simulink model "closed_loop_system_monitoring"  (R2025b)
settings: Solver=FixedStepAuto  StartTime=0.0  StopTime=2  RelTol=1e-3
values from neighbouring files (symbols this model uses):
  A = [Ac 0*Ac ... (first row only)    [closed_loop_system.m]
  B = [Bc ... (first row only)    [closed_loop_system.m]
  C = [0 0 Cp]    [closed_loop_system.m]
  Ts = 1/100    (= 0.01)    [closed_loop_system.m]
(part 1 of 2)
settings Model: NumberOfSteps=5  Creator=elia  LastModifiedBy=elia

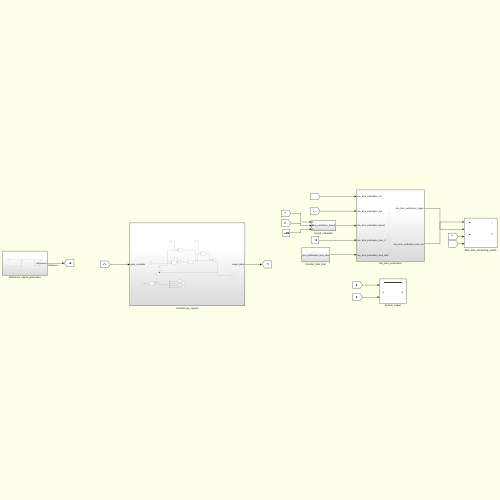
[thumbnail: Simulink's stored preview of the top-level diagram]
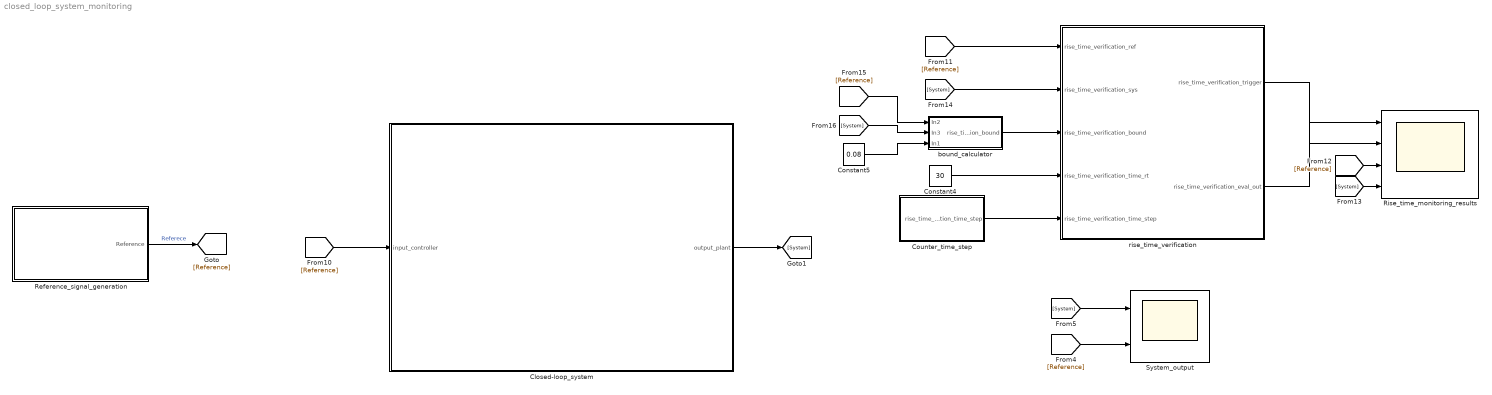
== system closed_loop_system_monitoring ==
  Closed-loop_system : Subsystem
  Constant4 : Constant  Value=30
  Constant5 : Constant  Value=0.08
  Counter_time_step : Subsystem
  Reference_signal_generation : Subsystem
  Rise_time_monitoring_results : Scope  NumInputPorts=4
      settings: ShowGrid=off  ActiveDisplayYMinimum=-0.12499999999999997  ActiveDisplayYMaximum=1.125  DataLoggingVariableName=ScopeData6
  System_output : Scope  NumInputPorts=2
      settings: ActiveDisplayYMinimum=-4.4796097220764581  ActiveDisplayYMaximum=1.9125014477904037
  bound_calculator : Subsystem
  rise_time_verification : Subsystem
  wires:
  Reference_signal_generation/1(Reference) -> [Reference]  "Referece"
  Closed-loop_system/1(output_plant) -> [System]
  [Reference] -> System_output/2
  [System] -> System_output/1
  [Reference] -> Closed-loop_system/1(input_controller)
  [System] -> rise_time_verification/2(rise_time_verification_sys)
  Constant4/1 -> rise_time_verification/4(rise_time_verification_time_rt)
  [System] -> Rise_time_monitoring_results/4
  rise_time_verification/2(rise_time_verification_eval_out) -> Rise_time_monitoring_results/1
  rise_time_verification/1(rise_time_verification_trigger) -> Rise_time_monitoring_results/2
  [Reference] -> Rise_time_monitoring_results/3
  Counter_time_step/1(rise_time_verification_time_step) -> rise_time_verification/5(rise_time_verification_time_step)
  [Reference] -> rise_time_verification/1(rise_time_verification_ref)
  Constant5/1 -> bound_calculator/3(In1)
  bound_calculator/1(rise_time_verification_bound) -> rise_time_verification/3(rise_time_verification_bound)
  [Reference] -> bound_calculator/1(In2)
  [System] -> bound_calculator/2(In3)

== system closed_loop_system_monitoring/Closed-loop_system ==
  input_controller : Inport
  Add : Sum  Inputs=-+
  Add1 : Sum
  Constant : Constant  Value=A
  Constant1 : Constant  Value=B
  Constant2 : Constant  Value=C
  Constant3 : Constant
  Constant4 : Constant  Value=0
  Constant5 : Constant  Value=0
  Constant6 : Constant  Value=0
  Matrix Multiply{,1..3} (4 alike) : Product  Multiplication=Matrix(*)
  Saturation : Subsystem
  Scope : Scope
  Transpose : Math  Operator=transpose
  Unit Delay : UnitDelay  SampleTime=-1  HasFrameUpgradeWarning=on
  Vector Concatenate : Concatenate  NumInputs=4
  output_plant : Outport
  wires:
  Constant/1 -> Matrix Multiply/1
  Constant1/1 -> Matrix Multiply1/1
  Saturation/1(Out1) -> Matrix Multiply1/2
  Add/1 -> Saturation/1(In1)
  Matrix Multiply2/1 -> Add/2
  Constant2/1 -> Matrix Multiply2/2
  Add1/1 -> Scope/1, Matrix Multiply3/2, Unit Delay/1
  Unit Delay/1 -> Matrix Multiply/2, Matrix Multiply2/1
  input_controller/1 -> Add/1
  Matrix Multiply1/1 -> Add1/1
  Matrix Multiply/1 -> Add1/2
  Vector Concatenate/1 -> Transpose/1
  Matrix Multiply3/1 -> output_plant/1
  Constant3/1 -> Vector Concatenate/3
  Constant4/1 -> Vector Concatenate/2
  Constant5/1 -> Vector Concatenate/1
  Constant6/1 -> Vector Concatenate/4
  Transpose/1 -> Matrix Multiply3/1

== system closed_loop_system_monitoring/Counter_time_step ==
  Add : Sum
  Constant4 : Constant  Value=0
  Constant5 : Constant
  Scope2 : Scope
      settings: ActiveDisplayYMinimum=-61.499999999999986  ActiveDisplayYMaximum=563.5  DataLoggingVariableName=ScopeData5
  Switch : Switch  Criteria=u2 ~= 0  SaturateOnIntegerOverflow=off  InputSameDT=off
  Unit Delay : UnitDelay  SampleTime=Ts  HasFrameUpgradeWarning=on
  Unit Delay1 : UnitDelay  SampleTime=Ts  HasFrameUpgradeWarning=on
  rise_time_verification_time_step : Outport
  wires:
  Switch/1 -> Add/1
  Add/1 -> Scope2/1, rise_time_verification_time_step/1, Unit Delay/1
  Constant5/1 -> Add/2
  Unit Delay1/1 -> Switch/2
  Unit Delay/1 -> Switch/3
  Constant4/1 -> Switch/1, Unit Delay1/1

== system closed_loop_system_monitoring/Reference_signal_generation ==
  Scope : Scope
      settings: ActiveDisplayYMinimum=0.9  ActiveDisplayYMaximum=1.1  DataLoggingVariableName=ScopeData4
  Step1 : Step  Time=0  Before=0.0  After=1.0  SampleTime=Ts
  Step2 : Step  Before=0.0  After=-3.0  SampleTime=Ts
  Sum : Sum  Inputs=|++
  Reference : Outport
  wires:
  Sum/1 -> Scope/1, Reference/1
  Step1/1 -> Sum/1  "input_1"
  Step2/1 -> Sum/2  "input_2"

== system closed_loop_system_monitoring/bound_calculator ==
  In2 : Inport
  In3 : Inport  Port=2
  In1 : Inport  Port=3
  Abs : Abs  SaturateOnIntegerOverflow=off
  Constant : Constant  Value=0
  Delay One Step : Delay  DelayLength=1  SampleTime=Ts
  Delay One Step1 : Delay  DelayLength=1  SampleTime=Ts
  Delay One Step2 : Delay  DelayLength=1  SampleTime=Ts
  Equal : RelationalOperator  Operator===  OutDataTypeStr=boolean  RndMeth=Simplest  InputSameDT=off
  NOT : Logic  Operator=NOT  IconShape=distinctive  AllPortsSameDT=off  OutDataTypeStr=boolean
  Product : Product
  Sum : Sum  Inputs=|+-
  Switch : Switch  Criteria=u2 > Threshold  SaturateOnIntegerOverflow=off  InputSameDT=off
  init : Switch  Criteria=u2 ~= 0  SaturateOnIntegerOverflow=off  InputSameDT=off
  rise_time_verification_bound : Outport
  wires:
  init/1 -> Delay One Step2/1, Product/1
  Constant/1 -> Delay One Step/1
  Delay One Step/1 -> init/2
  In2/1 -> Sum/1, Delay One Step1/1, Equal/1
  In3/1 -> Sum/2
  Sum/1 -> Abs/1
  Abs/1 -> Switch/1, init/1
  In1/1 -> Product/2
  Product/1 -> rise_time_verification_bound/1
  Equal/1 -> NOT/1
  NOT/1 -> Switch/2
  Delay One Step1/1 -> Equal/2
  Delay One Step2/1 -> Switch/3
  Switch/1 -> init/3

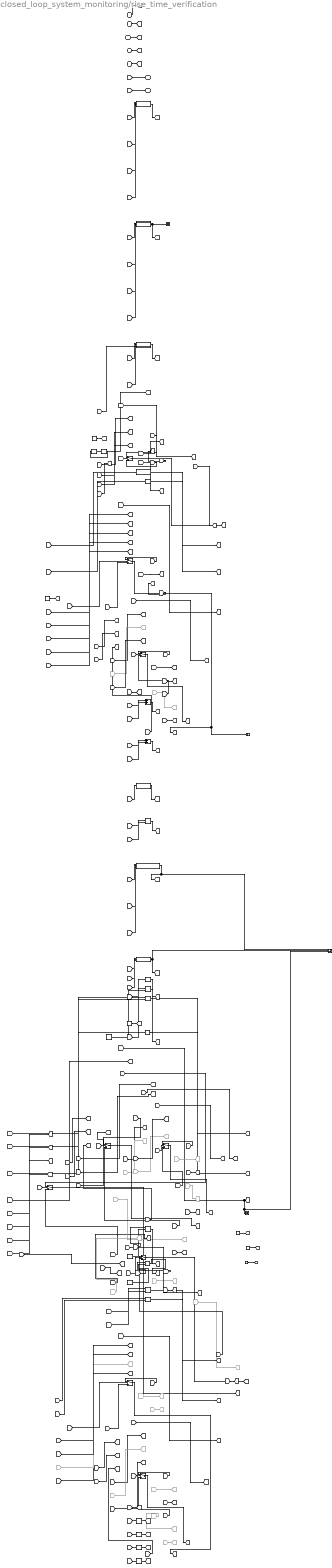
== system closed_loop_system_monitoring/rise_time_verification ==
  note: INIT time_step_reset
      | OK
  note: ITE time_step_reset
      | Guard+b_false OK
  note: ITE eval_out
      | OK
  note: INIT eval_out
      | Guard+init OK
  note: ITE eval : guard = pre trigger and pre eval
      | OK
  note: INIT trigger
      | OK
  note: ITE eval : guard = trigger
      | Guard+b_true OK
  note: ITE eval : guard = not ev_3v_T
      | OK
  note: ITE eval : guard = not ev_3v_F
      | OK
  rise_time_verification_ref : Inport  OutDataTypeStr=double
  rise_time_verification_sys : Inport  Port=2  OutDataTypeStr=double
  rise_time_verification_bound : Inport  Port=3  OutDataTypeStr=double
  rise_time_verification_time_rt : Inport  Port=4
  rise_time_verification_time_step : Inport  Port=5
  Arrow_xxrise_tim_1069005429_on_1_ni_18 : Delay  DelayLength=1  InitialCondition=1
  Constant : Constant  Value=0.5
  Constant1 : Constant  Value=1.0
  Constant2 : Constant  Value=0.25
  PRE_xxrise_time_verification_{2,11,13,22} (4 alike) : Delay  DelayLength=1  InitialCondition=0
  Scope : Scope
      settings: ActiveDisplayYMinimum=0.49776379028009476  ActiveDisplayYMaximum=0.51187913719672951  DataLoggingVariableName=ScopeData8
  Scope1 : Scope
      settings: ActiveDisplayYMinimum=-0.019336367279446723  ActiveDisplayYMaximum=0.04758303740367098  DataLoggingVariableName=ScopeData9
  Scope2 : Scope  NumInputPorts=3
      settings: ActiveDisplayYMinimum=-0.12499999999999997  ActiveDisplayYMaximum=1.125  DataLoggingVariableName=ScopeData10
  Scope3 : Scope
      settings: ActiveDisplayYMinimum=-50.249999999999986  ActiveDisplayYMaximum=452.25  DataLoggingVariableName=ScopeData11
  a_alse_xxrise_time_verification_7_out1 : Goto  Commented=on  GotoTag=a_alse_xxrise_time_verification_7
  a_alse_xxrise_time_verification_7_out2 : Goto  Commented=on  GotoTag=a_alse_xxrise_time_verification_7
  a_alse_xxrise_time_verification_7_out3 : Goto  Commented=on  GotoTag=a_alse_xxrise_time_verification_7
  a_lse_xxrise_time_verification_22_out1 : Goto  Commented=on  GotoTag=a_lse_xxrise_time_verification_22
  a_true_xxrise_time_verification_7_out{,1..2,4} (4 alike) : Goto  Commented=on  GotoTag=a_true_xxrise_time_verification_7
  absolute_value_call : Subsystem
  branch_13_IF : Switch  Criteria=u2 ~= 0  SaturateOnIntegerOverflow=off  InputSameDT=off
  branch_14_IF : Switch  Criteria=u2 ~= 0  SaturateOnIntegerOverflow=off  InputSameDT=off
  branch_15_IF : Switch  Criteria=u2 ~= 0  SaturateOnIntegerOverflow=off  InputSameDT=off
  branch_15_In2 : From  Commented=on  GotoTag=a_lse_xxrise_time_verification_22
  branch_15_branch_false_In1 : From  Commented=on  GotoTag=branch_15_xxrise_time_verification_22
  branch_15_xxrise_time_verification_22_out : Goto  Commented=on  GotoTag=branch_15_xxrise_time_verification_22
  branch_16_IF : Switch  Criteria=u2 ~= 0  SaturateOnIntegerOverflow=off  InputSameDT=off
  branch_17_IF : Switch  Criteria=u2 ~= 0  SaturateOnIntegerOverflow=off  InputSameDT=off
  branch_17_branch_false_In1 : From  Commented=on  GotoTag=branch_17_xxrise_time_verification_7
  branch_17_branch_true_In2 : From  Commented=on  GotoTag=branch_17_xxrise_time_verification_7
  branch_18_IF : Switch  Criteria=u2 ~= 0  SaturateOnIntegerOverflow=off  InputSameDT=off
  branch_18_In2 : From  Commented=on  GotoTag=a_true_xxrise_time_verification_7
  branch_18_branch_false_In1 : From  Commented=on  GotoTag=branch_18_xxrise_time_verification_7
  branch_18_branch_true_In1 : From  Commented=on  GotoTag=branch_18_xxrise_time_verification_7
  branch_18_xxrise_time_verification_7_out : Goto  Commented=on  GotoTag=branch_18_xxrise_time_verification_7
  branch_19_IF : Switch  Criteria=u2 ~= 0  SaturateOnIntegerOverflow=off  InputSameDT=off
  branch_19_In2 : From  Commented=on  GotoTag=a_alse_xxrise_time_verification_7
  branch_19_branch_false_In1 : From  Commented=on  GotoTag=branch_19_xxrise_time_verification_7
  branch_19_branch_true_In1 : From  Commented=on  GotoTag=branch_19_xxrise_time_verification_7
  branch_19_xxrise_time_verification_7_out : Goto  Commented=on  GotoTag=branch_19_xxrise_time_verification_7
  branch_20_IF : Switch  Criteria=u2 ~= 0  SaturateOnIntegerOverflow=off  InputSameDT=off
  branch_20_In3 : From  Commented=on  GotoTag=a_tion_xxrise_time_verification_7
  branch_20_branch_true_In1 : From  Commented=on  GotoTag=branch_20_eval
  branch_20_branch_true_eval_out : Goto  Commented=on  GotoTag=branch_20_branch_true_eval
  branch_20_xxrise_time_verification_7_out : Goto  Commented=on  GotoTag=branch_20_xxrise_time_verification_7
  branch_21_IF : Switch  Criteria=u2 ~= 0  SaturateOnIntegerOverflow=off  InputSameDT=off
  branch_21_In2 : From  Commented=on  GotoTag=a_alse_xxrise_time_verification_7
  branch_21_branch_false_In1 : From  Commented=on  GotoTag=branch_21_eval
  branch_21_branch_false_eval_out : Goto  Commented=on  GotoTag=branch_21_branch_false_eval
  branch_21_branch_true_In1 : From  Commented=on  GotoTag=branch_21_xxrise_time_verification_7
  branch_21_xxrise_time_verification_7_out : Goto  Commented=on  GotoTag=branch_21_xxrise_time_verification_7
  condition_R_call : Subsystem
  eventually_false_var_call : Subsystem
  eventually_true_var_call : Subsystem
  trigger_general_rt_call : Subsystem
  trigger_off_rise_time_call : Subsystem
  trigger_on_rise_time_call : Subsystem
  xxrise_tim_1069005429_on_1_ni_18_init : Constant  Value=0  OutDataTypeStr=boolean
  xxrise_time_verification_10_operator : Logic  Operator=NOT  AllPortsSameDT=off  OutDataTypeStr=boolean
  xxrise_time_verification_12_operator : RelationalOperator  Operator===  OutDataTypeStr=boolean  RndMeth=Simplest  InputSameDT=off
  xxrise_time_verification_12_rhs_2 : Constant  Value=0.5  OutDataTypeStr=double
  xxrise_time_verification_14_operator : Logic  AllPortsSameDT=off  OutDataTypeStr=boolean
  xxrise_time_verification_15_operator : Sum  Inputs=+-  OutDataTypeStr=double
  xxrise_time_verification_17_operator : RelationalOperator  Operator=<=  OutDataTypeStr=boolean  RndMeth=Simplest  InputSameDT=off
  xxrise_time_verification_18_operator : Sum  OutDataTypeStr=int32
  xxrise_time_verification_19_rhs : Constant  Value=0  OutDataTypeStr=Inherit: Inherit via back propagation
  xxrise_time_verification_21_operator : Logic  Operator=NOT  AllPortsSameDT=off  OutDataTypeStr=boolean
  xxrise_time_verification_24_rhs : Constant  Value=false  OutDataTypeStr=boolean
  xxrise_time_verification_3_operator : RelationalOperator  Operator===  OutDataTypeStr=boolean  RndMeth=Simplest  InputSameDT=off
  xxrise_time_verification_3_rhs_2 : Constant  Value=0.0  OutDataTypeStr=double
  xxrise_time_verification_4_operator : RelationalOperator  Operator===  OutDataTypeStr=boolean  RndMeth=Simplest  InputSameDT=off
  xxrise_time_verification_4_rhs_2 : Constant  Value=0.0  OutDataTypeStr=double
  xxrise_time_verification_5_operator : Logic  Operator=OR  AllPortsSameDT=off  OutDataTypeStr=boolean
  xxrise_time_verification_6_operator : Logic  AllPortsSameDT=off  OutDataTypeStr=boolean
  xxrise_time_verification_7_rhs : Constant  Value=0.0  OutDataTypeStr=double
  xxrise_time_verification_8_lhs : Goto  Commented=on  GotoTag=a_alse_xxrise_time_verification_8
  xxrise_time_verification_8_lhs2 : Goto  Commented=on  GotoTag=a_true_xxrise_time_verification_8
  xxrise_time_verification_8_rhs : From  Commented=on  GotoTag=branch_21_branch_false_eval
  xxrise_time_verification_8_rhs2 : From  Commented=on  GotoTag=branch_20_branch_true_eval
  xxrise_time_verification_9_operator : Logic  Operator=NOT  AllPortsSameDT=off  OutDataTypeStr=boolean
  rise_time_verification_trigger : Outport
  rise_time_verification_eval_out : Outport  Port=2
  wires:
  rise_time_verification_ref/1 -> [rise_time_verification_ref]
  rise_time_verification_sys/1 -> [rise_time_verification_sys]
  rise_time_verification_bound/1 -> [rise_time_verification_bound]
  rise_time_verification_time_rt/1 -> [rise_time_verification_time_rt]
  rise_time_verification_time_step/1 -> [rise_time_verification_time_step]
  [rise_time_verification_trigger] -> rise_time_verification_trigger/1
  [rise_time_verification_eval_out] -> rise_time_verification_eval_out/1
  trigger_on_rise_time_call/1(trigger_on_rise_time_trigger) -> [rise_time_verification_ev_ON]
  [a_ion_xxrise_time_verification_13] -> trigger_on_rise_time_call/1(trigger_on_rise_time_p_trigger)
  [rise_time_verification_ref] -> trigger_on_rise_time_call/2(trigger_on_rise_time_ref)
  [rise_time_verification_sys] -> trigger_on_rise_time_call/3(trigger_on_rise_time_sys)
  [rise_time_verification_bound] -> trigger_on_rise_time_call/4(trigger_on_rise_time_bound)
  trigger_off_rise_time_call/1(trigger_off_rise_time_trigger) -> [rise_time_verification_ev_OFF], Scope1/1
  [a_ion_xxrise_time_verification_13] -> trigger_off_rise_time_call/1(trigger_off_rise_time_p_trigger)
  [rise_time_verification_ref] -> trigger_off_rise_time_call/2(trigger_off_rise_time_ref)
  [rise_time_verification_sys] -> trigger_off_rise_time_call/3(trigger_off_rise_time_sys)
  [rise_time_verification_bound] -> trigger_off_rise_time_call/4(trigger_off_rise_time_bound)
  trigger_general_rt_call/1(trigger_general_rt_trigger_out) -> [a_ion_xxrise_time_verification_25]
  [rise_time_verification_ev_ON] -> trigger_general_rt_call/1(trigger_general_rt_ev_ON)
  [rise_time_verification_ev_OFF] -> trigger_general_rt_call/2(trigger_general_rt_ev_OFF)
  [rise_time_verification_ref] -> trigger_general_rt_call/3(trigger_general_rt_r)
  xxrise_time_verification_24_rhs/1 -> [a_ion_xxrise_time_verification_24]
  xxrise_tim_1069005429_on_1_ni_18_init/1 -> Arrow_xxrise_tim_1069005429_on_1_ni_18/1
  Arrow_xxrise_tim_1069005429_on_1_ni_18/1 -> [a_tion_xxrise_time_verification_1]
  [branch_13_xxrise_time_verification_26] -> [a_ion_xxrise_time_verification_26]
  branch_13_IF/1 -> [branch_13_xxrise_time_verification_26]
  [a_lse_xxrise_time_verification_26] -> branch_13_IF/3
  [a_rue_xxrise_time_verification_26] -> branch_13_IF/1
  [branch_13_xxrise_time_verification_1] -> branch_13_IF/2
  [a_ion_xxrise_time_verification_25] -> [branch_13_xxrise_time_verification_25]
  [a_ion_xxrise_time_verification_24] -> [branch_13_xxrise_time_verification_24]
  [a_tion_xxrise_time_verification_1] -> [branch_13_xxrise_time_verification_1]
  [a_lse_xxrise_time_verification_25] -> [a_lse_xxrise_time_verification_26]
  [branch_13_xxrise_time_verification_25] -> [a_lse_xxrise_time_verification_25]
  [a_rue_xxrise_time_verification_24] -> [a_rue_xxrise_time_verification_26]
  [branch_13_xxrise_time_verification_24] -> [a_rue_xxrise_time_verification_24]
  [a_ion_xxrise_time_verification_26] -> [rise_time_verification_trigger]
  condition_R_call/1(condition_R_const_deriv) -> [a_ion_xxrise_time_verification_20]
  [rise_time_verification_ref] -> condition_R_call/1(condition_R_r)
  xxrise_time_verification_21_operator/1 -> [a_ion_xxrise_time_verification_21]
  [a_ion_xxrise_time_verification_20] -> xxrise_time_verification_21_operator/1
  xxrise_time_verification_19_rhs/1 -> [a_ion_xxrise_time_verification_19]
  [branch_14_xxrise_time_verification_23] -> [a_ion_xxrise_time_verification_23]
  branch_14_IF/1 -> Scope3/1, [branch_14_xxrise_time_verification_23]
  [a_lse_xxrise_time_verification_23_b_14_in] -> branch_14_IF/3
  [a_rue_xxrise_time_verification_23_b_14_init] -> branch_14_IF/1
  [branch_14_xxrise_time_verification_1] -> branch_14_IF/2
  [rise_time_verification_time_step] -> [branch_14_time_step]
  [a_ion_xxrise_time_verification_22] -> [branch_14_xxrise_time_verification_22]
  [a_ion_xxrise_time_verification_21] -> [branch_14_xxrise_time_verification_21]
  [a_ion_xxrise_time_verification_19] -> [branch_14_xxrise_time_verification_19]
  [a_tion_xxrise_time_verification_1] -> [branch_14_xxrise_time_verification_1]
  [branch_15_time_step] -> [branch_15_branch_true_time_step]
  [branch_15_branch_true_time_step] -> [a_rue_xxrise_time_verification_23]
  branch_15_branch_false_In1/1 -> a_lse_xxrise_time_verification_22_out1/1
  [a_lse_xxrise_time_verification_22_b_15_f] -> [a_lse_xxrise_time_verification_23]
  [a_lse_xxrise_time_verification_21] -> [branch_15_xxrise_time_verification_21]
  branch_15_In2/1 -> branch_15_xxrise_time_verification_22_out/1
  [branch_14_branch_false_time_step] -> [branch_15_time_step]
  [branch_15_xxrise_time_verification_21] -> branch_15_IF/2
  [a_rue_xxrise_time_verification_23] -> branch_15_IF/1
  [a_lse_xxrise_time_verification_23] -> branch_15_IF/3
  branch_15_IF/1 -> [branch_15_xxrise_time_verification_23]
  [branch_15_xxrise_time_verification_23] -> [a_lse_xxrise_time_verification_23_b_14_in]
  [branch_14_time_step] -> [branch_14_branch_false_time_step]
  [branch_14_xxrise_time_verification_22] -> [a_lse_xxrise_time_verification_22_b_15_f]
  [branch_14_xxrise_time_verification_21] -> [a_lse_xxrise_time_verification_21]
  [a_rue_xxrise_time_verification_19] -> [a_rue_xxrise_time_verification_23_b_14_init]
  [branch_14_xxrise_time_verification_19] -> [a_rue_xxrise_time_verification_19]
  [a_ion_xxrise_time_verification_23] -> [rise_time_verification_time_step_reset]
  xxrise_time_verification_18_operator/1 -> [a_ion_xxrise_time_verification_18]
  [rise_time_verification_time_rt] -> xxrise_time_verification_18_operator/1
  [rise_time_verification_time_step_reset] -> xxrise_time_verification_18_operator/2
  xxrise_time_verification_15_operator/1 -> [a_ion_xxrise_time_verification_15]
  [rise_time_verification_sys] -> xxrise_time_verification_15_operator/1
  [rise_time_verification_ref] -> xxrise_time_verification_15_operator/2
  absolute_value_call/1(absolute_value_abs) -> [a_ion_xxrise_time_verification_16]
  [a_ion_xxrise_time_verification_15] -> absolute_value_call/1(absolute_value_x)
  xxrise_time_verification_17_operator/1 -> [a_ion_xxrise_time_verification_17]
  [a_ion_xxrise_time_verification_16] -> xxrise_time_verification_17_operator/1
  [rise_time_verification_bound] -> xxrise_time_verification_17_operator/2
  eventually_true_var_call/1(eventually_true_var_output_ev_true) -> [rise_time_verification_eventually_3v_T], Scope2/1
  [rise_time_verification_time_step_reset] -> eventually_true_var_call/1(eventually_true_var_a)
  [a_ion_xxrise_time_verification_18] -> eventually_true_var_call/2(eventually_true_var_b)
  [a_ion_xxrise_time_verification_17] -> eventually_true_var_call/3(eventually_true_var_phi)
  eventually_false_var_call/1(eventually_false_var_output_ev_false) -> Scope2/2, [rise_time_verification_eventually_3v_F]
  [rise_time_verification_time_step_reset] -> eventually_false_var_call/1(eventually_false_var_a)
  [a_ion_xxrise_time_verification_18] -> eventually_false_var_call/2(eventually_false_var_b)
  [a_ion_xxrise_time_verification_17] -> eventually_false_var_call/3(eventually_false_var_phi)
  xxrise_time_verification_9_operator/1 -> [a_tion_xxrise_time_verification_9]
  [rise_time_verification_eventually_3v_T] -> xxrise_time_verification_9_operator/1
  xxrise_time_verification_7_rhs/1 -> [a_tion_xxrise_time_verification_7]
  xxrise_time_verification_12_operator/1 -> [a_ion_xxrise_time_verification_12]
  [a_ion_xxrise_time_verification_11] -> xxrise_time_verification_12_operator/1
  xxrise_time_verification_12_rhs_2/1 -> xxrise_time_verification_12_operator/2
  xxrise_time_verification_14_operator/1 -> [a_ion_xxrise_time_verification_14]
  [a_ion_xxrise_time_verification_13] -> xxrise_time_verification_14_operator/1
  [a_ion_xxrise_time_verification_12] -> xxrise_time_verification_14_operator/2
  xxrise_time_verification_10_operator/1 -> [a_ion_xxrise_time_verification_10]
  [rise_time_verification_eventually_3v_F] -> xxrise_time_verification_10_operator/1
  [branch_16_eval] -> Scope2/3, Scope/1, [rise_time_verification_eval]
  branch_16_IF/1 -> [branch_16_eval]
  [branch_16_branch_false_eval] -> branch_16_IF/3
  [branch_16_branch_true_eval] -> branch_16_IF/1
  [branch_16_trigger] -> branch_16_IF/2
  [rise_time_verification_trigger] -> [branch_16_trigger]
  [a_tion_xxrise_time_verification_9] -> [branch_16_xxrise_time_verification_9]
  [a_tion_xxrise_time_verification_7] -> [branch_16_xxrise_time_verification_7]
  [a_ion_xxrise_time_verification_14] -> [branch_16_xxrise_time_verification_14]
  [a_ion_xxrise_time_verification_10] -> [branch_16_xxrise_time_verification_10]
  branch_19_branch_true_In1/1 -> a_true_xxrise_time_verification_7_out/1
  [const_1_0] -> [branch_19_branch_true_eval]
  branch_19_branch_false_In1/1 -> a_alse_xxrise_time_verification_7_out1/1
  [a_alse_xxrise_time_verification_7] -> [branch_19_branch_false_eval]
  [a_lse_xxrise_time_verification_14] -> [branch_19_xxrise_time_verification_14]
  branch_19_In2/1 -> branch_19_xxrise_time_verification_7_out/1
  [branch_19_xxrise_time_verification_14] -> branch_19_IF/2
  [branch_19_branch_true_eval] -> branch_19_IF/1
  [branch_19_branch_false_eval] -> branch_19_IF/3
  branch_19_IF/1 -> [branch_19_eval]
  [branch_19_eval] -> [branch_16_branch_false_eval]
  [branch_16_xxrise_time_verification_7] -> [a_alse_xxrise_time_verification_7_b_18_F]
  [branch_16_xxrise_time_verification_14] -> [a_lse_xxrise_time_verification_14]
  [branch_17_xxrise_time_verification_10] -> [a_rue_xxrise_time_verification_10]
  branch_17_branch_true_In2/1 -> a_true_xxrise_time_verification_7_out2/1
  [branch_18_eval] -> [branch_17_branch_true_eval]
  branch_18_IF/1 -> [branch_18_eval]
  [branch_18_branch_false_eval] -> branch_18_IF/3
  [branch_18_branch_true_eval] -> branch_18_IF/1
  [branch_18_xxrise_time_verification_10] -> branch_18_IF/2
  branch_18_In2/1 -> branch_18_xxrise_time_verification_7_out/1
  [a_rue_xxrise_time_verification_10] -> [branch_18_xxrise_time_verification_10]
  [a_alse_xxrise_time_verification_7_b_18_F] -> [branch_18_branch_false_eval]
  branch_18_branch_false_In1/1 -> a_alse_xxrise_time_verification_7_out3/1
  [const_0_5] -> [branch_18_branch_true_eval]
  branch_18_branch_true_In1/1 -> a_true_xxrise_time_verification_7_out1/1
  branch_17_branch_false_In1/1 -> a_alse_xxrise_time_verification_7_out2/1
  [const_1_0] -> [branch_17_branch_false_eval]
  [a_rue_xxrise_time_verification_10_guard_b_18] -> [branch_17_xxrise_time_verification_10]
  [a_true_xxrise_time_verification_7] -> [branch_17_xxrise_time_verification_7]
  [a_true_xxrise_time_verification_9] -> [branch_17_xxrise_time_verification_9]
  [branch_17_xxrise_time_verification_9] -> branch_17_IF/2
  [branch_17_branch_true_eval] -> branch_17_IF/1
  [branch_17_branch_false_eval] -> branch_17_IF/3
  branch_17_IF/1 -> [branch_17_eval]
  [branch_17_eval] -> [branch_16_branch_true_eval]
  [branch_16_xxrise_time_verification_9] -> [a_true_xxrise_time_verification_9]
  [branch_16_xxrise_time_verification_7] -> [a_true_xxrise_time_verification_7]
  [branch_16_xxrise_time_verification_10] -> [a_rue_xxrise_time_verification_10_guard_b_18]
  xxrise_time_verification_4_operator/1 -> [a_tion_xxrise_time_verification_4]
  [rise_time_verification_eval] -> xxrise_time_verification_4_operator/1
  xxrise_time_verification_4_rhs_2/1 -> xxrise_time_verification_4_operator/2
  xxrise_time_verification_3_operator/1 -> [a_tion_xxrise_time_verification_3]
  [a_tion_xxrise_time_verification_2] -> xxrise_time_verification_3_operator/1
  xxrise_time_verification_3_rhs_2/1 -> xxrise_time_verification_3_operator/2
  xxrise_time_verification_5_operator/1 -> [a_tion_xxrise_time_verification_5]
  [a_tion_xxrise_time_verification_4] -> xxrise_time_verification_5_operator/1
  [a_tion_xxrise_time_verification_3] -> xxrise_time_verification_5_operator/2
  xxrise_time_verification_6_operator/1 -> [a_tion_xxrise_time_verification_6]
  [rise_time_verification_trigger] -> xxrise_time_verification_6_operator/1
  [a_tion_xxrise_time_verification_5] -> xxrise_time_verification_6_operator/2
  [branch_20_xxrise_time_verification_8] -> [a_tion_xxrise_time_verification_8]
  branch_20_IF/1 -> [branch_20_xxrise_time_verification_8]
  [a_alse_xxrise_time_verification_8_b_21_F] -> branch_20_IF/3
  [rise_time_verification_eval] -> branch_20_IF/1
  [branch_20_xxrise_time_verification_1] -> branch_20_IF/2
  [rise_time_verification_eval] -> [branch_20_eval]
  branch_20_In3/1 -> branch_20_xxrise_time_verification_7_out/1
  [a_tion_xxrise_time_verification_6] -> [branch_20_xxrise_time_verification_6]
  [a_tion_xxrise_time_verification_1] -> [branch_20_xxrise_time_verification_1]
  branch_21_branch_true_In1/1 -> a_true_xxrise_time_verification_7_out4/1
  [a_true_xxrise_time_verification_7] -> [a_true_xxrise_time_verification_8_b_21_in]
  branch_21_branch_false_In1/1 -> branch_21_branch_false_eval_out/1
  xxrise_time_verification_8_rhs/1 -> xxrise_time_verification_8_lhs/1
  [a_alse_xxrise_time_verification_6] -> [branch_21_xxrise_time_verification_6]
  branch_21_In2/1 -> branch_21_xxrise_time_verification_7_out/1
  [branch_20_branch_false_eval] -> [branch_21_eval]
  [branch_21_xxrise_time_verification_6] -> branch_21_IF/2
  [a_true_xxrise_time_verification_8_b_21_in] -> branch_21_IF/1
  [rise_time_verification_eval] -> branch_21_IF/3
  branch_21_IF/1 -> [branch_21_xxrise_time_verification_8]
  [branch_21_xxrise_time_verification_8] -> [a_alse_xxrise_time_verification_8_b_21_F]
  [branch_20_eval] -> [branch_20_branch_false_eval]
  [const_0_25] -> [a_alse_xxrise_time_verification_7]
  [branch_20_xxrise_time_verification_6] -> [a_alse_xxrise_time_verification_6]
  xxrise_time_verification_8_rhs2/1 -> xxrise_time_verification_8_lhs2/1
  branch_20_branch_true_In1/1 -> branch_20_branch_true_eval_out/1
  [a_tion_xxrise_time_verification_8] -> [rise_time_verification_eval_out]
  [rise_time_verification_time_step_reset] -> PRE_xxrise_time_verification_22/1
  PRE_xxrise_time_verification_22/1 -> [a_ion_xxrise_time_verification_22]
  [rise_time_verification_eval_out] -> PRE_xxrise_time_verification_2/1
  PRE_xxrise_time_verification_2/1 -> [a_tion_xxrise_time_verification_2]
  [rise_time_verification_trigger] -> PRE_xxrise_time_verification_13/1
  PRE_xxrise_time_verification_13/1 -> [a_ion_xxrise_time_verification_13]
  [rise_time_verification_eval] -> PRE_xxrise_time_verification_11/1
  PRE_xxrise_time_verification_11/1 -> [a_ion_xxrise_time_verification_11]
  Constant/1 -> [const_0_5]
  Constant1/1 -> [const_1_0]
  Constant2/1 -> [const_0_25]

== system closed_loop_system_monitoring/Closed-loop_system/Saturation ==
  In1 : Inport
  Constant : Constant  Value=1.0
  Constant1 : Constant  Value=-1.0
  Switch : Switch  Criteria=u2 > Threshold  Threshold=1.0  SaturateOnIntegerOverflow=off  InputSameDT=off
  Switch1 : Switch  Criteria=u2 > Threshold  Threshold=-1.0  SaturateOnIntegerOverflow=off  InputSameDT=off
  Out1 : Outport
  wires:
  Constant1/1 -> Switch1/3
  Constant/1 -> Switch/1
  Switch/1 -> Switch1/2, Switch1/1
  Switch1/1 -> Out1/1
  In1/1 -> Switch/2, Switch/3

== system closed_loop_system_monitoring/rise_time_verification/absolute_value_call ==
  absolute_value_x : Inport  OutDataTypeStr=double
  branch_8_IF : Switch  Criteria=u2 ~= 0  SaturateOnIntegerOverflow=off  InputSameDT=off
  xxabsolute_value_1_operator : RelationalOperator  OutDataTypeStr=boolean  RndMeth=Simplest  InputSameDT=off
  xxabsolute_value_1_rhs_2 : Constant  Value=0.0  OutDataTypeStr=double
  xxabsolute_value_2_operator : Gain  Gain=-1  OutDataTypeStr=double
  absolute_value_abs : Outport
  wires:
  [branch_8_x] -> [branch_8_branch_true_x]
  [branch_8_branch_true_x] -> [branch_8_branch_true_abs]
  [branch_8_xxabsolute_value_2] -> [branch_8_branch_false_xxabsolute_value_2]
  [branch_8_branch_false_xxabsolute_value_2] -> [branch_8_branch_false_abs]
  [absolute_value_xxabsolute_value_1] -> [branch_8_xxabsolute_value_1]
  [absolute_value_xxabsolute_value_2] -> [branch_8_xxabsolute_value_2]
  [absolute_value_x] -> [branch_8_x]
  [branch_8_xxabsolute_value_1] -> branch_8_IF/2
  [branch_8_branch_true_abs] -> branch_8_IF/1
  [branch_8_branch_false_abs] -> branch_8_IF/3
  branch_8_IF/1 -> [branch_8_abs]
  [branch_8_abs] -> [absolute_value_abs]
  xxabsolute_value_1_rhs_2/1 -> xxabsolute_value_1_operator/2
  [absolute_value_x] -> xxabsolute_value_1_operator/1
  xxabsolute_value_1_operator/1 -> [absolute_value_xxabsolute_value_1]
  [absolute_value_x] -> xxabsolute_value_2_operator/1
  xxabsolute_value_2_operator/1 -> [absolute_value_xxabsolute_value_2]
  [absolute_value_abs] -> absolute_value_abs/1
  absolute_value_x/1 -> [absolute_value_x]

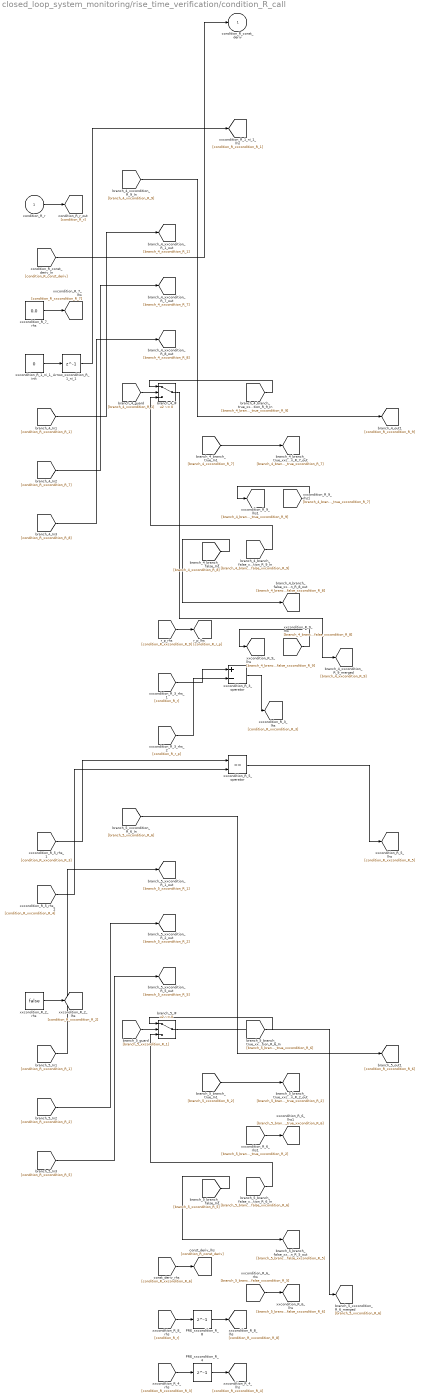
== system closed_loop_system_monitoring/rise_time_verification/condition_R_call ==
  condition_R_r : Inport  OutDataTypeStr=double
  Arrow_xxcondition_R_1_ni_1 : Delay  DelayLength=1  InitialCondition=1
  PRE_xxcondition_R_4 : Delay  DelayLength=1  InitialCondition=0
  PRE_xxcondition_R_8 : Delay  DelayLength=1  InitialCondition=0
  branch_4_IF : Switch  Criteria=u2 ~= 0  SaturateOnIntegerOverflow=off  InputSameDT=off
  branch_5_IF : Switch  Criteria=u2 ~= 0  SaturateOnIntegerOverflow=off  InputSameDT=off
  xxcondition_R_1_ni_1_init : Constant  Value=0  OutDataTypeStr=boolean
  xxcondition_R_2_rhs : Constant  Value=false  OutDataTypeStr=boolean
  xxcondition_R_3_operator : Sum  Inputs=+-  OutDataTypeStr=double
  xxcondition_R_5_operator : RelationalOperator  Operator===  OutDataTypeStr=boolean  RndMeth=Simplest  InputSameDT=off
  xxcondition_R_7_rhs : Constant  Value=0.0  OutDataTypeStr=double
  condition_R_const_deriv : Outport
  wires:
  PRE_xxcondition_R_4/1 -> [condition_R_xxcondition_R_4]
  [condition_R_xxcondition_R_3] -> PRE_xxcondition_R_4/1
  PRE_xxcondition_R_8/1 -> [condition_R_xxcondition_R_8]
  [condition_R_r] -> PRE_xxcondition_R_8/1
  [condition_R_xxcondition_R_6] -> [condition_R_const_deriv]
  [branch_5_xxcondition_R_2] -> [branch_5_branch_true_xxcondition_R_2]
  [branch_5_branch_true_xxcondition_R_2] -> [branch_5_branch_true_xxcondition_R_6]
  [branch_5_xxcondition_R_5] -> [branch_5_branch_false_xxcondition_R_5]
  [branch_5_branch_false_xxcondition_R_5] -> [branch_5_branch_false_xxcondition_R_6]
  [condition_R_xxcondition_R_1] -> [branch_5_xxcondition_R_1]
  [condition_R_xxcondition_R_2] -> [branch_5_xxcondition_R_2]
  [condition_R_xxcondition_R_5] -> [branch_5_xxcondition_R_5]
  [branch_5_xxcondition_R_1] -> branch_5_IF/2
  [branch_5_branch_true_xxcondition_R_6] -> branch_5_IF/1
  [branch_5_branch_false_xxcondition_R_6] -> branch_5_IF/3
  branch_5_IF/1 -> [branch_5_xxcondition_R_6]
  [branch_5_xxcondition_R_6] -> [condition_R_xxcondition_R_6]
  xxcondition_R_2_rhs/1 -> [condition_R_xxcondition_R_2]
  [condition_R_xxcondition_R_4] -> xxcondition_R_5_operator/2
  [condition_R_xxcondition_R_3] -> xxcondition_R_5_operator/1
  xxcondition_R_5_operator/1 -> [condition_R_xxcondition_R_5]
  [condition_R_r_p] -> xxcondition_R_3_operator/2
  [condition_R_r] -> xxcondition_R_3_operator/1
  xxcondition_R_3_operator/1 -> [condition_R_xxcondition_R_3]
  [condition_R_xxcondition_R_9] -> [condition_R_r_p]
  [branch_4_xxcondition_R_7] -> [branch_4_branch_true_xxcondition_R_7]
  [branch_4_branch_true_xxcondition_R_7] -> [branch_4_branch_true_xxcondition_R_9]
  [branch_4_xxcondition_R_8] -> [branch_4_branch_false_xxcondition_R_8]
  [branch_4_branch_false_xxcondition_R_8] -> [branch_4_branch_false_xxcondition_R_9]
  [condition_R_xxcondition_R_1] -> [branch_4_xxcondition_R_1]
  [condition_R_xxcondition_R_7] -> [branch_4_xxcondition_R_7]
  [condition_R_xxcondition_R_8] -> [branch_4_xxcondition_R_8]
  [branch_4_xxcondition_R_1] -> branch_4_IF/2
  [branch_4_branch_true_xxcondition_R_9] -> branch_4_IF/1
  [branch_4_branch_false_xxcondition_R_9] -> branch_4_IF/3
  branch_4_IF/1 -> [branch_4_xxcondition_R_9]
  [branch_4_xxcondition_R_9] -> [condition_R_xxcondition_R_9]
  Arrow_xxcondition_R_1_ni_1/1 -> [condition_R_xxcondition_R_1]
  xxcondition_R_1_ni_1_init/1 -> Arrow_xxcondition_R_1_ni_1/1
  xxcondition_R_7_rhs/1 -> [condition_R_xxcondition_R_7]
  [condition_R_const_deriv] -> condition_R_const_deriv/1
  condition_R_r/1 -> [condition_R_r]

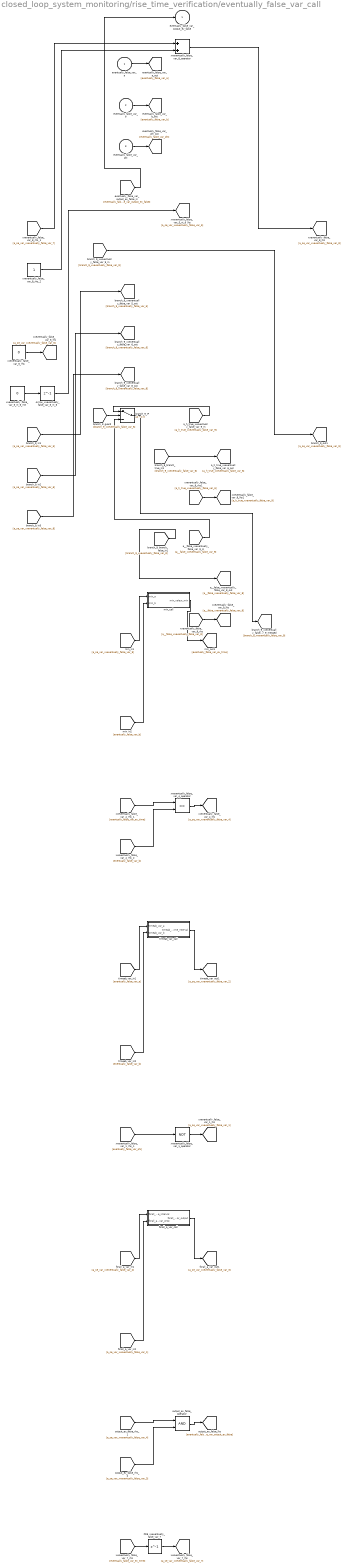
== system closed_loop_system_monitoring/rise_time_verification/eventually_false_var_call ==
  eventually_false_var_a : Inport
  eventually_false_var_b : Inport  Port=2
  eventually_false_var_phi : Inport  Port=3  OutDataTypeStr=boolean
  Arrow_xxeventually_false_var_5_ni_6 : Delay  DelayLength=1  InitialCondition=1
  PRE_xxeventually_false_var_7 : Delay  DelayLength=1  InitialCondition=0
  branch_9_IF : Switch  Criteria=u2 ~= 0  SaturateOnIntegerOverflow=off  InputSameDT=off
  forall_a_var_call : Subsystem
  min_call : Subsystem
  output_ev_false_operator : Logic  AllPortsSameDT=off  OutDataTypeStr=boolean
  timeab_var_call : Subsystem
  xxeventually_false_var_1_operator : Logic  Operator=NOT  AllPortsSameDT=off  OutDataTypeStr=boolean
  xxeventually_false_var_4_operator : RelationalOperator  Operator===  OutDataTypeStr=boolean  RndMeth=Simplest  InputSameDT=off
  xxeventually_false_var_5_ni_6_init : Constant  Value=0  OutDataTypeStr=boolean
  xxeventually_false_var_6_rhs : Constant  Value=0  OutDataTypeStr=Inherit: Inherit via back propagation
  xxeventually_false_var_8_operator : Sum  OutDataTypeStr=int32
  xxeventually_false_var_8_rhs_2 : Constant  OutDataTypeStr=int32
  eventually_false_var_output_ev_false : Outport
  wires:
  PRE_xxeventually_false_var_7/1 -> [a_se_var_xxeventually_false_var_7]
  [eventually_false_var_ev_time] -> PRE_xxeventually_false_var_7/1
  [a_se_var_xxeventually_false_var_3] -> output_ev_false_operator/2
  [a_se_var_xxeventually_false_var_4] -> output_ev_false_operator/1
  output_ev_false_operator/1 -> [eventually_false_var_output_ev_false]
  [a_se_var_xxeventually_false_var_1] -> forall_a_var_call/2(forall_a_var_prop)
  [a_se_var_xxeventually_false_var_2] -> forall_a_var_call/1(forall_a_var_inside_time_interval)
  forall_a_var_call/1(forall_a_var_output) -> [a_se_var_xxeventually_false_var_3]
  [eventually_false_var_phi] -> xxeventually_false_var_1_operator/1
  xxeventually_false_var_1_operator/1 -> [a_se_var_xxeventually_false_var_1]
  [eventually_false_var_b] -> timeab_var_call/2(timeab_var_b)
  [eventually_false_var_a] -> timeab_var_call/1(timeab_var_a)
  timeab_var_call/1(timeab_var_inside_time_interval) -> [a_se_var_xxeventually_false_var_2]
  [eventually_false_var_b] -> xxeventually_false_var_4_operator/2
  [eventually_false_var_ev_time] -> xxeventually_false_var_4_operator/1
  xxeventually_false_var_4_operator/1 -> [a_se_var_xxeventually_false_var_4]
  [eventually_false_var_b] -> min_call/2(min_b)
  [a_se_var_xxeventually_false_var_9] -> min_call/1(min_a)
  min_call/1(min_valeur_min) -> [eventually_false_var_ev_time]
  [branch_9_xxeventually_false_var_6] -> [a_h_true_xxeventually_false_var_6]
  [a_h_true_xxeventually_false_var_6] -> [a_h_true_xxeventually_false_var_9]
  [branch_9_xxeventually_false_var_8] -> [a__false_xxeventually_false_var_8]
  [a__false_xxeventually_false_var_8] -> [a__false_xxeventually_false_var_9]
  [a_se_var_xxeventually_false_var_5] -> [branch_9_xxeventually_false_var_5]
  [a_se_var_xxeventually_false_var_6] -> [branch_9_xxeventually_false_var_6]
  [a_se_var_xxeventually_false_var_8] -> [branch_9_xxeventually_false_var_8]
  [branch_9_xxeventually_false_var_5] -> branch_9_IF/2
  [a_h_true_xxeventually_false_var_9] -> branch_9_IF/1
  [a__false_xxeventually_false_var_9] -> branch_9_IF/3
  branch_9_IF/1 -> [branch_9_xxeventually_false_var_9]
  [branch_9_xxeventually_false_var_9] -> [a_se_var_xxeventually_false_var_9]
  Arrow_xxeventually_false_var_5_ni_6/1 -> [a_se_var_xxeventually_false_var_5]
  xxeventually_false_var_5_ni_6_init/1 -> Arrow_xxeventually_false_var_5_ni_6/1
  xxeventually_false_var_6_rhs/1 -> [a_se_var_xxeventually_false_var_6]
  xxeventually_false_var_8_rhs_2/1 -> xxeventually_false_var_8_operator/2
  [a_se_var_xxeventually_false_var_7] -> xxeventually_false_var_8_operator/1
  xxeventually_false_var_8_operator/1 -> [a_se_var_xxeventually_false_var_8]
  [eventually_false_var_output_ev_false] -> eventually_false_var_output_ev_false/1
  eventually_false_var_phi/1 -> [eventually_false_var_phi]
  eventually_false_var_b/1 -> [eventually_false_var_b]
  eventually_false_var_a/1 -> [eventually_false_var_a]

== system closed_loop_system_monitoring/rise_time_verification/eventually_true_var_call ==
  eventually_true_var_a : Inport
  eventually_true_var_b : Inport  Port=2
  eventually_true_var_phi : Inport  Port=3  OutDataTypeStr=boolean
  exist_var_call : Subsystem
  timeab_var_call : Subsystem
  eventually_true_var_output_ev_true : Outport
  wires:
  [eventually_true_var_phi] -> exist_var_call/2(exist_var_prop)
  [eventually_true_var_xxeventually_true_var_1] -> exist_var_call/1(exist_var_inside_time_interval)
  exist_var_call/1(exist_var_output) -> [eventually_true_var_output_ev_true]
  [eventually_true_var_b] -> timeab_var_call/2(timeab_var_b)
  [eventually_true_var_a] -> timeab_var_call/1(timeab_var_a)
  timeab_var_call/1(timeab_var_inside_time_interval) -> [eventually_true_var_xxeventually_true_var_1]
  [eventually_true_var_output_ev_true] -> eventually_true_var_output_ev_true/1
  eventually_true_var_phi/1 -> [eventually_true_var_phi]
  eventually_true_var_b/1 -> [eventually_true_var_b]
  eventually_true_var_a/1 -> [eventually_true_var_a]

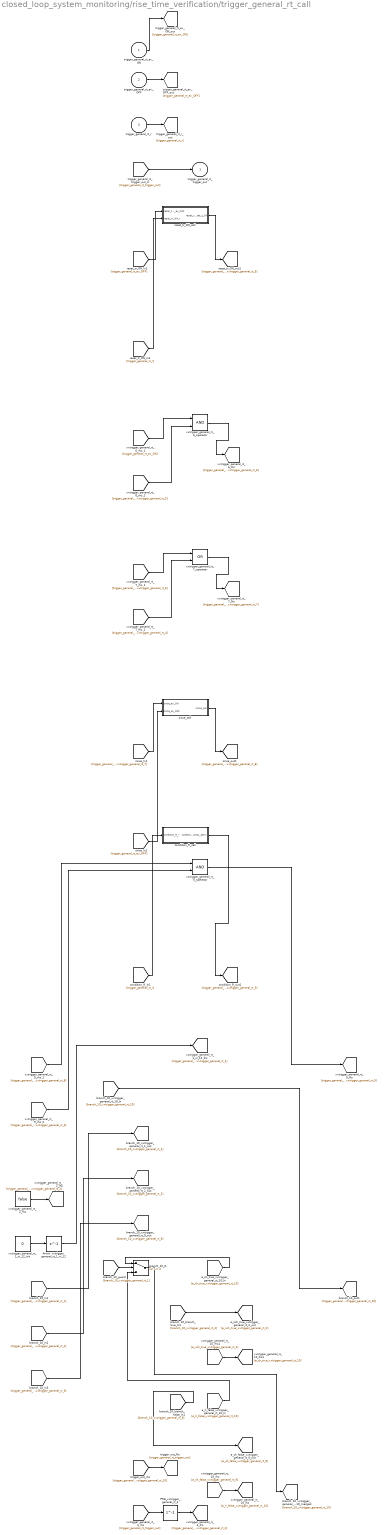
== system closed_loop_system_monitoring/rise_time_verification/trigger_general_rt_call ==
  trigger_general_rt_ev_ON : Inport  OutDataTypeStr=boolean
  trigger_general_rt_ev_OFF : Inport  Port=2  OutDataTypeStr=boolean
  trigger_general_rt_r : Inport  Port=3  OutDataTypeStr=double
  Arrow_xxtrigger_general_rt_1_ni_12 : Delay  DelayLength=1  InitialCondition=1
  PRE_xxtrigger_general_rt_4 : Delay  DelayLength=1  InitialCondition=0
  branch_10_IF : Switch  Criteria=u2 ~= 0  SaturateOnIntegerOverflow=off  InputSameDT=off
  condition_R_call : Subsystem
  reset_tr_ON_call : Subsystem
  since_call : Subsystem
  xxtrigger_general_rt_1_ni_12_init : Constant  Value=0  OutDataTypeStr=boolean
  xxtrigger_general_rt_2_rhs : Constant  Value=false  OutDataTypeStr=boolean
  xxtrigger_general_rt_6_operator : Logic  AllPortsSameDT=off  OutDataTypeStr=boolean
  xxtrigger_general_rt_7_operator : Logic  Operator=OR  AllPortsSameDT=off  OutDataTypeStr=boolean
  xxtrigger_general_rt_9_operator : Logic  AllPortsSameDT=off  OutDataTypeStr=boolean
  trigger_general_rt_trigger_out : Outport
  wires:
  PRE_xxtrigger_general_rt_4/1 -> [trigger_general_rt_xxtrigger_general_rt_4]
  [trigger_general_rt_trigger_out] -> PRE_xxtrigger_general_rt_4/1
  [trigger_general_rt_xxtrigger_general_rt_10] -> [trigger_general_rt_trigger_out]
  [branch_10_xxtrigger_general_rt_2] -> [a_nch_true_xxtrigger_general_rt_2]
  [a_nch_true_xxtrigger_general_rt_2] -> [a_ch_true_xxtrigger_general_rt_10]
  [branch_10_xxtrigger_general_rt_9] -> [a_ch_false_xxtrigger_general_rt_9]
  [a_ch_false_xxtrigger_general_rt_9] -> [a_h_false_xxtrigger_general_rt_10]
  [trigger_general_rt_xxtrigger_general_rt_1] -> [branch_10_xxtrigger_general_rt_1]
  [trigger_general_rt_xxtrigger_general_rt_2] -> [branch_10_xxtrigger_general_rt_2]
  [trigger_general_rt_xxtrigger_general_rt_9] -> [branch_10_xxtrigger_general_rt_9]
  [branch_10_xxtrigger_general_rt_1] -> branch_10_IF/2
  [a_ch_true_xxtrigger_general_rt_10] -> branch_10_IF/1
  [a_h_false_xxtrigger_general_rt_10] -> branch_10_IF/3
  branch_10_IF/1 -> [branch_10_xxtrigger_general_rt_10]
  [branch_10_xxtrigger_general_rt_10] -> [trigger_general_rt_xxtrigger_general_rt_10]
  Arrow_xxtrigger_general_rt_1_ni_12/1 -> [trigger_general_rt_xxtrigger_general_rt_1]
  xxtrigger_general_rt_1_ni_12_init/1 -> Arrow_xxtrigger_general_rt_1_ni_12/1
  xxtrigger_general_rt_2_rhs/1 -> [trigger_general_rt_xxtrigger_general_rt_2]
  [trigger_general_rt_xxtrigger_general_rt_3] -> xxtrigger_general_rt_9_operator/2
  [trigger_general_rt_xxtrigger_general_rt_8] -> xxtrigger_general_rt_9_operator/1
  xxtrigger_general_rt_9_operator/1 -> [trigger_general_rt_xxtrigger_general_rt_9]
  [trigger_general_rt_r] -> condition_R_call/1(condition_R_r)
  condition_R_call/1(condition_R_const_deriv) -> [trigger_general_rt_xxtrigger_general_rt_3]
  [trigger_general_rt_ev_OFF] -> since_call/2(since_ev_OFF)
  [trigger_general_rt_xxtrigger_general_rt_7] -> since_call/1(since_ev_ON)
  since_call/1(since_out) -> [trigger_general_rt_xxtrigger_general_rt_8]
  [trigger_general_rt_xxtrigger_general_rt_4] -> xxtrigger_general_rt_7_operator/2
  [trigger_general_rt_xxtrigger_general_rt_6] -> xxtrigger_general_rt_7_operator/1
  xxtrigger_general_rt_7_operator/1 -> [trigger_general_rt_xxtrigger_general_rt_7]
  [trigger_general_rt_xxtrigger_general_rt_5] -> xxtrigger_general_rt_6_operator/2
  [trigger_general_rt_ev_ON] -> xxtrigger_general_rt_6_operator/1
  xxtrigger_general_rt_6_operator/1 -> [trigger_general_rt_xxtrigger_general_rt_6]
  [trigger_general_rt_r] -> reset_tr_ON_call/2(reset_tr_ON_r)
  [trigger_general_rt_ev_OFF] -> reset_tr_ON_call/1(reset_tr_ON_ev_OFF)
  reset_tr_ON_call/1(reset_tr_ON_reset_t_ON) -> [trigger_general_rt_xxtrigger_general_rt_5]
  [trigger_general_rt_trigger_out] -> trigger_general_rt_trigger_out/1
  trigger_general_rt_r/1 -> [trigger_general_rt_r]
  trigger_general_rt_ev_OFF/1 -> [trigger_general_rt_ev_OFF]
  trigger_general_rt_ev_ON/1 -> [trigger_general_rt_ev_ON]

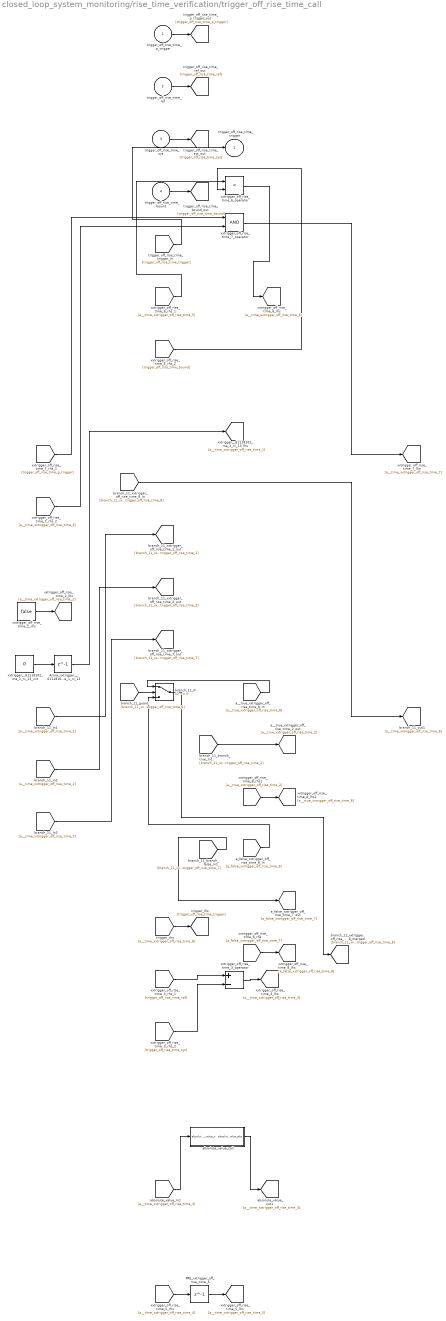
== system closed_loop_system_monitoring/rise_time_verification/trigger_off_rise_time_call ==
  trigger_off_rise_time_p_trigger : Inport  OutDataTypeStr=boolean
  trigger_off_rise_time_ref : Inport  Port=2  OutDataTypeStr=double
  trigger_off_rise_time_sys : Inport  Port=3  OutDataTypeStr=double
  trigger_off_rise_time_bound : Inport  Port=4  OutDataTypeStr=double
  Arrow_xxtrigger__61118102_me_1_ni_13 : Delay  DelayLength=1  InitialCondition=1
  PRE_xxtrigger_off_rise_time_5 : Delay  DelayLength=1  InitialCondition=0
  absolute_value_call : Subsystem
  branch_11_IF : Switch  Criteria=u2 ~= 0  SaturateOnIntegerOverflow=off  InputSameDT=off
  xxtrigger__61118102_me_1_ni_13_init : Constant  Value=0  OutDataTypeStr=boolean
  xxtrigger_off_rise_time_2_rhs : Constant  Value=false  OutDataTypeStr=boolean
  xxtrigger_off_rise_time_3_operator : Sum  Inputs=+-  OutDataTypeStr=double
  xxtrigger_off_rise_time_6_operator : RelationalOperator  Operator=<  OutDataTypeStr=boolean  RndMeth=Simplest  InputSameDT=off
  xxtrigger_off_rise_time_7_operator : Logic  AllPortsSameDT=off  OutDataTypeStr=boolean
  trigger_off_rise_time_trigger : Outport
  wires:
  PRE_xxtrigger_off_rise_time_5/1 -> [a__time_xxtrigger_off_rise_time_5]
  [a__time_xxtrigger_off_rise_time_4] -> PRE_xxtrigger_off_rise_time_5/1
  [a__time_xxtrigger_off_rise_time_3] -> absolute_value_call/1(absolute_value_x)
  absolute_value_call/1(absolute_value_abs) -> [a__time_xxtrigger_off_rise_time_4]
  [trigger_off_rise_time_sys] -> xxtrigger_off_rise_time_3_operator/2
  [trigger_off_rise_time_ref] -> xxtrigger_off_rise_time_3_operator/1
  xxtrigger_off_rise_time_3_operator/1 -> [a__time_xxtrigger_off_rise_time_3]
  [a__time_xxtrigger_off_rise_time_8] -> [trigger_off_rise_time_trigger]
  [branch_11_xxtrigger_off_rise_time_2] -> [a__true_xxtrigger_off_rise_time_2]
  [a__true_xxtrigger_off_rise_time_2] -> [a__true_xxtrigger_off_rise_time_8]
  [branch_11_xxtrigger_off_rise_time_7] -> [a_false_xxtrigger_off_rise_time_7]
  [a_false_xxtrigger_off_rise_time_7] -> [a_false_xxtrigger_off_rise_time_8]
  [a__time_xxtrigger_off_rise_time_1] -> [branch_11_xxtrigger_off_rise_time_1]
  [a__time_xxtrigger_off_rise_time_2] -> [branch_11_xxtrigger_off_rise_time_2]
  [a__time_xxtrigger_off_rise_time_7] -> [branch_11_xxtrigger_off_rise_time_7]
  [branch_11_xxtrigger_off_rise_time_1] -> branch_11_IF/2
  [a__true_xxtrigger_off_rise_time_8] -> branch_11_IF/1
  [a_false_xxtrigger_off_rise_time_8] -> branch_11_IF/3
  branch_11_IF/1 -> [branch_11_xxtrigger_off_rise_time_8]
  [branch_11_xxtrigger_off_rise_time_8] -> [a__time_xxtrigger_off_rise_time_8]
  Arrow_xxtrigger__61118102_me_1_ni_13/1 -> [a__time_xxtrigger_off_rise_time_1]
  xxtrigger__61118102_me_1_ni_13_init/1 -> Arrow_xxtrigger__61118102_me_1_ni_13/1
  xxtrigger_off_rise_time_2_rhs/1 -> [a__time_xxtrigger_off_rise_time_2]
  [a__time_xxtrigger_off_rise_time_6] -> xxtrigger_off_rise_time_7_operator/2
  [trigger_off_rise_time_p_trigger] -> xxtrigger_off_rise_time_7_operator/1
  xxtrigger_off_rise_time_7_operator/1 -> [a__time_xxtrigger_off_rise_time_7]
  [trigger_off_rise_time_bound] -> xxtrigger_off_rise_time_6_operator/2
  [a__time_xxtrigger_off_rise_time_5] -> xxtrigger_off_rise_time_6_operator/1
  xxtrigger_off_rise_time_6_operator/1 -> [a__time_xxtrigger_off_rise_time_6]
  [trigger_off_rise_time_trigger] -> trigger_off_rise_time_trigger/1
  trigger_off_rise_time_bound/1 -> [trigger_off_rise_time_bound]
  trigger_off_rise_time_sys/1 -> [trigger_off_rise_time_sys]
  trigger_off_rise_time_ref/1 -> [trigger_off_rise_time_ref]
  trigger_off_rise_time_p_trigger/1 -> [trigger_off_rise_time_p_trigger]
